simulink model "MagneticIp_model"  (R2024b)
settings: Solver=FixedStepAuto  StartTime=0.0  StopTime=10.0  RelTol=1e-3
settings Model: Creator=felipe  LastModifiedBy=felipe
settings OptimizationCC: PassReuseOutputArgsAs=Individual arguments  OptimizeBlockOrder=speed  DifferentSizesBufferReuse=on  EfficientTunableParamExpr=on
settings DebuggingCC: ParameterTunabilityLossMsg=error
settings HardwareCC: TargetBitPerLong=64  TargetBitPerPointer=64  TargetBitPerSizeT=64  TargetBitPerPtrDiffT=64  TargetLongLongMode=on  TargetIntDivRoundTo=Zero  TargetEndianess=LittleEndian  TargetWordSize=64  TargetHWDeviceType=MATLAB Host  ProdEqTarget=off
settings SFSimCC: MATLABDynamicMemAlloc=off
settings RTWCC: Description=Embedded Coder (host-based shared library target)  SystemTargetFile=ert_shrlib.tlc  TemplateMakefile=ert_default_tmf  RTWVerbose=off
settings RTWCC: CustomSourceCode=|
  | #define CONCAT(str1, str2, str3) CONCAT_(str1, str2, str3)
  | #define CONCAT_(str1, str2, str3) str1 ## str2 ## str3
  | #define GET_MMI_FUNC    CONCAT(MODEL     , _GetCAPImmi ,    )
  | #define RT_MODEL_STRUCT CONCAT(RT_MODEL_ , MODEL       , _T )
  | 
  | void* GET_MMI_FUNC(void* voidPtrToRealTimeStructure)
  | {
  |    rtwCAPI_ModelMappingInfo* mmiPtr = &(rtmGetDataMapInfo( ( RT_MODEL_STRUCT * )(voidPtrToRealTimeStructure) ).mmi);
  |    return (void*) mmiPtr;
  | }
settings CodeAppCC: GenerateComments=off  IgnoreCustomStorageClasses=off  OperatorAnnotations=on  SimulinkDataObjDesc=on  SFDataObjDesc=on  SimulinkBlockComments=off
settings STFCustomTargetCC: TargetLangStandard=C99 (ISO)  MultiwordLength=256  ParMdlRefBuildCompliant=on  CompOptLevelCompliant=on  IncludeMdlTerminateFcn=off  CombineOutputUpdateFcns=on  CombineSignalStateStructs=on  SuppressErrorStatus=on  ERTCustomFileBanners=on  SupportAbsoluteTime=off  CodeInterfacePackaging=Reusable function  SupportComplex=off  SupportContinuousTime=off  SupportNonInlinedSFcns=off  RemoveResetFunc=on  MATLABClassNameForMDSCustomization=Simulink.SoftwareTarget.ERTCustomization  ModelStepFunctionPrototypeControlCompliant=on  GenerateAllocFcn=on  UseToolchainInfoCompliant=on  SystemTargetFile=ert_shrlib.tlc
settings ERTTargetCC: TargetLangStandard=C99 (ISO)  ConcurrentExecutionCompliant=off  IncludeMdlTerminateFcn=off  CombineSignalStateStructs=on  SuppressErrorStatus=on  SupportAbsoluteTime=off  CodeInterfacePackaging=Reusable function  SupportComplex=off  CPPClassGenCompliant=off  GenerateAllocFcn=on  InlinedParameterPlacement=Hierarchical  RootIOFormat=Part of model data structure  RTWCAPIParams=on  RTWCAPIRootIO=on  ERTCustomFileTemplate=example_file_process.tlc

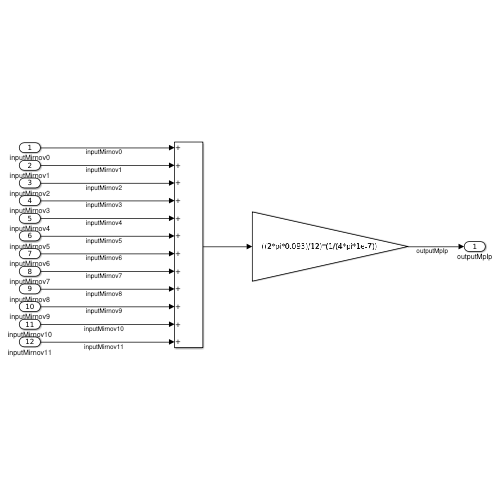
[thumbnail: Simulink's stored preview of the top-level diagram]
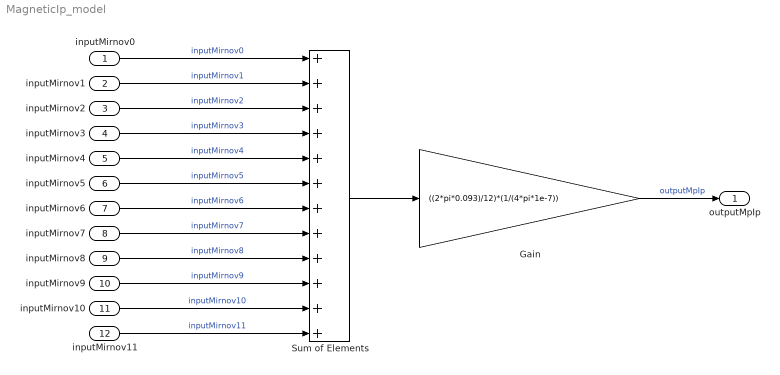
== system MagneticIp_model ==
  inputMirnov0 : Inport  OutDataTypeStr=double
  inputMirnov1 : Inport  Port=2  OutDataTypeStr=double
  inputMirnov2 : Inport  Port=3  OutDataTypeStr=double
  inputMirnov3 : Inport  Port=4  OutDataTypeStr=double
  inputMirnov4 : Inport  Port=5  OutDataTypeStr=double
  inputMirnov5 : Inport  Port=6  OutDataTypeStr=double
  inputMirnov6 : Inport  Port=7  OutDataTypeStr=double
  inputMirnov7 : Inport  Port=8  OutDataTypeStr=double
  inputMirnov8 : Inport  Port=9  OutDataTypeStr=double
  inputMirnov9 : Inport  Port=10  OutDataTypeStr=double
  inputMirnov10 : Inport  Port=11  OutDataTypeStr=double
  inputMirnov11 : Inport  Port=12  OutDataTypeStr=double
  Gain : Gain  Gain=((2*pi*0.093)/12)*(1/(4*pi*1e-7))
  Sum of Elements : Sum  Inputs=++++++++++++
  outputMpIp : Outport  OutDataTypeStr=double
  wires:
  inputMirnov5/1 -> Sum of Elements/6  "inputMirnov5"
  inputMirnov4/1 -> Sum of Elements/5  "inputMirnov4"
  inputMirnov0/1 -> Sum of Elements/1  "inputMirnov0"
  inputMirnov11/1 -> Sum of Elements/12  "inputMirnov11"
  inputMirnov10/1 -> Sum of Elements/11  "inputMirnov10"
  inputMirnov9/1 -> Sum of Elements/10  "inputMirnov9"
  inputMirnov8/1 -> Sum of Elements/9  "inputMirnov8"
  inputMirnov7/1 -> Sum of Elements/8  "inputMirnov7"
  inputMirnov6/1 -> Sum of Elements/7  "inputMirnov6"
  inputMirnov1/1 -> Sum of Elements/2  "inputMirnov1"
  inputMirnov2/1 -> Sum of Elements/3  "inputMirnov2"
  inputMirnov3/1 -> Sum of Elements/4  "inputMirnov3"
  Sum of Elements/1 -> Gain/1
  Gain/1 -> outputMpIp/1  "outputMpIp"
